simulink model "HANcoder_E407_TTA_Controller_v4_5"  (R2018b)
settings: Solver=FixedStepDiscrete  StartTime=0.0  StopTime=1  FixedStep=0.01  RelTol=1e-3
PreLoadFcn:
  | librarySetup
  | eval([bdroot,'_startup']) %Calling [modelName]_startup.m
values from neighbouring files (symbols this model uses):
  Backup_Board = 0    [HANcoder_E407_TTA_Controller_v3_5_startup.m]    (also in HANcoder_E407_TTA_Controller_v4_6_startup.m; HANcoder_E407_TTA_Controller_v4_7_startup.m; HANcoder_E407_TTA_Controller_v4_startup.m)
  basic_cycle_duration_bc0 = TM_Reset_Board   + COMP_duration    (= 212)    [HANcoder_E407_TTA_Controller_v3_5_startup.m]    (also in HANcoder_E407_TTA_Controller_v4_6_startup.m; HANcoder_E407_TTA_Controller_v4_7_startup.m; HANcoder_E407_TTA_Controller_v4_startup.m)
  basic_cycle_duration_bc1 = TM_Reset_Var_bc1 + COMP_duration    (= 288)    [HANcoder_E407_TTA_Controller_v3_5_startup.m]    (also in HANcoder_E407_TTA_Controller_v4_6_startup.m = 332; HANcoder_E407_TTA_Controller_v4_7_startup.m = 372; HANcoder_E407_TTA_Controller_v4_startup.m = 332)
  comm_delay_estimation1 = round(comm_delay_measured1*hardware_granularity/frequency_IRQ)    [HANcoder_E407_TTA_Controller_v3_5_startup.m]    (also in HANcoder_E407_TTA_Controller_v4_6_startup.m; HANcoder_E407_TTA_Controller_v4_7_startup.m; HANcoder_E407_TTA_Controller_v4_startup.m)
  comm_delay_estimation2 = round(comm_delay_measured2*hardware_granularity/frequency_IRQ)    [HANcoder_E407_TTA_Controller_v3_5_startup.m]    (also in HANcoder_E407_TTA_Controller_v4_6_startup.m; HANcoder_E407_TTA_Controller_v4_7_startup.m; HANcoder_E407_TTA_Controller_v4_startup.m)
  COMM_Period = 40    [HANcoder_E407_TTA_Controller_v3_5_startup.m]    (also in HANcoder_E407_TTA_Controller_v4_6_startup.m; HANcoder_E407_TTA_Controller_v4_7_startup.m; HANcoder_E407_TTA_Controller_v4_startup.m)
  COMM_Phase1 = Simulink.Parameter    [HANcoder_E407_TTA_Controller_v3_5_startup.m]    (also in HANcoder_E407_TTA_Controller_v4_6_startup.m; HANcoder_E407_TTA_Controller_v4_7_startup.m; HANcoder_E407_TTA_Controller_v4_startup.m)
  COMM_Phase2 = Simulink.Parameter    [HANcoder_E407_TTA_Controller_v3_5_startup.m]    (also in HANcoder_E407_TTA_Controller_v4_6_startup.m; HANcoder_E407_TTA_Controller_v4_7_startup.m; HANcoder_E407_TTA_Controller_v4_startup.m)
  COMM_Phase_init1 = Simulink.Parameter    [HANcoder_E407_TTA_Controller_v3_5_startup.m]    (also in HANcoder_E407_TTA_Controller_v4_6_startup.m; HANcoder_E407_TTA_Controller_v4_7_startup.m; HANcoder_E407_TTA_Controller_v4_startup.m)
  COMM_Phase_init2 = Simulink.Parameter    [HANcoder_E407_TTA_Controller_v3_5_startup.m]    (also in HANcoder_E407_TTA_Controller_v4_6_startup.m; HANcoder_E407_TTA_Controller_v4_7_startup.m; HANcoder_E407_TTA_Controller_v4_startup.m)
  COMP_duration = 4    [HANcoder_E407_TTA_Controller_v3_5_startup.m]    (also in HANcoder_E407_TTA_Controller_v4_6_startup.m; HANcoder_E407_TTA_Controller_v4_7_startup.m; HANcoder_E407_TTA_Controller_v4_startup.m)
  Controller1_Board = 1    [HANcoder_E407_TTA_Controller_v3_5_startup.m]    (also in HANcoder_E407_TTA_Controller_v4_6_startup.m; HANcoder_E407_TTA_Controller_v4_7_startup.m; HANcoder_E407_TTA_Controller_v4_startup.m)
  Controller2_Board = 2    [HANcoder_E407_TTA_Controller_v3_5_startup.m]    (also in HANcoder_E407_TTA_Controller_v4_6_startup.m; HANcoder_E407_TTA_Controller_v4_7_startup.m; HANcoder_E407_TTA_Controller_v4_startup.m)
  Controller3_Board = 3    [HANcoder_E407_TTA_Controller_v3_5_startup.m]    (also in HANcoder_E407_TTA_Controller_v4_6_startup.m; HANcoder_E407_TTA_Controller_v4_7_startup.m; HANcoder_E407_TTA_Controller_v4_startup.m)
  delta_a_set = Simulink.Parameter    [HANcoder_E407_TTA_Controller_v3_5_startup.m]    (also in HANcoder_E407_TTA_Controller_v4_6_startup.m; HANcoder_E407_TTA_Controller_v4_7_startup.m; HANcoder_E407_TTA_Controller_v4_startup.m)
  delta_f_set = Simulink.Parameter    [HANcoder_E407_TTA_Controller_v3_5_startup.m]    (also in HANcoder_E407_TTA_Controller_v4_6_startup.m; HANcoder_E407_TTA_Controller_v4_7_startup.m; HANcoder_E407_TTA_Controller_v4_startup.m)
  delta_max = 1    [HANcoder_E407_TTA_Controller_v3_5_startup.m]    (also in HANcoder_E407_TTA_Controller_v4_6_startup.m; HANcoder_E407_TTA_Controller_v4_7_startup.m; HANcoder_E407_TTA_Controller_v4_startup.m)
  delta_min = -1    [HANcoder_E407_TTA_Controller_v3_5_startup.m]    (also in HANcoder_E407_TTA_Controller_v4_6_startup.m; HANcoder_E407_TTA_Controller_v4_7_startup.m; HANcoder_E407_TTA_Controller_v4_startup.m)
  delta_precision = 6    [HANcoder_E407_TTA_Controller_v3_5_startup.m]    (also in HANcoder_E407_TTA_Controller_v4_6_startup.m; HANcoder_E407_TTA_Controller_v4_7_startup.m; HANcoder_E407_TTA_Controller_v4_startup.m)
  e_width = 0.1    [HANcoder_E407_TTA_Controller_v3_5_startup.m]    (also in HANcoder_E407_TTA_Controller_v4_6_startup.m; HANcoder_E407_TTA_Controller_v4_7_startup.m; HANcoder_E407_TTA_Controller_v4_startup.m)
  frequency_IRQ = 100    [HANcoder_E407_2xCAN_TEST_startup.m]    (also in HANcoder_E407_TTA_Controller_v3_5_startup.m; HANcoder_E407_TTA_Controller_v4_6_startup.m; HANcoder_E407_TTA_Controller_v4_7_startup.m; HANcoder_E407_TTA_Controller_v4_startup.m)
  HANtuneOverride = Simulink.Parameter    [HANcoder_E407_2xCAN_TEST_startup.m]    (also in HANcoder_E407_TTA_Controller_v3_5_startup.m; HANcoder_E407_TTA_Controller_v4_6_startup.m; HANcoder_E407_TTA_Controller_v4_7_startup.m; HANcoder_E407_TTA_Controller_v4_startup.m)
  hardware_granularity = 1000000    [HANcoder_E407_2xCAN_TEST_startup.m]    (also in HANcoder_E407_TTA_Controller_v3_5_startup.m; HANcoder_E407_TTA_Controller_v4_6_startup.m; HANcoder_E407_TTA_Controller_v4_7_startup.m; HANcoder_E407_TTA_Controller_v4_startup.m)
  I_a = 2.25    [HANcoder_E407_TTA_Controller_v3_5_startup.m]    (also in HANcoder_E407_TTA_Controller_v4_6_startup.m; HANcoder_E407_TTA_Controller_v4_7_startup.m; HANcoder_E407_TTA_Controller_v4_startup.m)
  I_f = 2.25    [HANcoder_E407_TTA_Controller_v3_5_startup.m]    (also in HANcoder_E407_TTA_Controller_v4_6_startup.m; HANcoder_E407_TTA_Controller_v4_7_startup.m; HANcoder_E407_TTA_Controller_v4_startup.m)
  idle_time_init = basic_cycle_duration_bc0 + basic_cycle_duration_bc1    (= 500)    [HANcoder_E407_TTA_Controller_v3_5_startup.m]    (also in HANcoder_E407_TTA_Controller_v4_6_startup.m = 544; HANcoder_E407_TTA_Controller_v4_7_startup.m = 584; HANcoder_E407_TTA_Controller_v4_startup.m = 544)
  Input_Gen_Board = 4    [HANcoder_E407_TTA_Controller_v3_5_startup.m]    (also in HANcoder_E407_TTA_Controller_v4_6_startup.m; HANcoder_E407_TTA_Controller_v4_7_startup.m; HANcoder_E407_TTA_Controller_v4_startup.m)
  LA_Clock_Gr = 1    [HANcoder_E407_TTA_Controller_v3_5_startup.m]    (also in HANcoder_E407_TTA_Controller_v4_6_startup.m; HANcoder_E407_TTA_Controller_v4_7_startup.m; HANcoder_E407_TTA_Controller_v4_startup.m)
  LA_COMM_dly = 1    [HANcoder_E407_TTA_Controller_v3_5_startup.m]    (also in HANcoder_E407_TTA_Controller_v4_6_startup.m; HANcoder_E407_TTA_Controller_v4_7_startup.m; HANcoder_E407_TTA_Controller_v4_startup.m)
  LA_COMM_Err = 1    [HANcoder_E407_TTA_Controller_v3_5_startup.m]    (also in HANcoder_E407_TTA_Controller_v4_6_startup.m; HANcoder_E407_TTA_Controller_v4_7_startup.m; HANcoder_E407_TTA_Controller_v4_startup.m)
  LA_E_Desync = 1    [HANcoder_E407_TTA_Controller_v3_5_startup.m]    (also in HANcoder_E407_TTA_Controller_v4_6_startup.m; HANcoder_E407_TTA_Controller_v4_7_startup.m; HANcoder_E407_TTA_Controller_v4_startup.m)
  LA_MEX_Flag = 1    [HANcoder_E407_TTA_Controller_v3_5_startup.m]    (also in HANcoder_E407_TTA_Controller_v4_6_startup.m; HANcoder_E407_TTA_Controller_v4_7_startup.m; HANcoder_E407_TTA_Controller_v4_startup.m)
  LA_Task_Act = 1    [HANcoder_E407_TTA_Controller_v3_5_startup.m]    (also in HANcoder_E407_TTA_Controller_v4_6_startup.m; HANcoder_E407_TTA_Controller_v4_7_startup.m; HANcoder_E407_TTA_Controller_v4_startup.m)
  m_v = 100.0    (= 100)    [HANcoder_E407_TTA_Controller_v3_5_startup.m]    (also in HANcoder_E407_TTA_Controller_v4_6_startup.m; HANcoder_E407_TTA_Controller_v4_7_startup.m; HANcoder_E407_TTA_Controller_v4_startup.m)
  Master_Role = 1    [HANcoder_E407_TTA_Controller_v3_5_startup.m]    (also in HANcoder_E407_TTA_Controller_v4_6_startup.m; HANcoder_E407_TTA_Controller_v4_7_startup.m; HANcoder_E407_TTA_Controller_v4_startup.m)
  matrix_cycle_duration = basic_cycle_duration_bc0 + basic_cycle_duration_bc1    (= 500)    [HANcoder_E407_TTA_Controller_v3_5_startup.m]    (also in HANcoder_E407_TTA_Controller_v4_6_startup.m = 544; HANcoder_E407_TTA_Controller_v4_7_startup.m = 584; HANcoder_E407_TTA_Controller_v4_startup.m = 544)
  matrix_rows = 2    [HANcoder_E407_TTA_Controller_v3_5_startup.m]    (also in HANcoder_E407_TTA_Controller_v4_6_startup.m; HANcoder_E407_TTA_Controller_v4_7_startup.m; HANcoder_E407_TTA_Controller_v4_startup.m)
  max_desync = 15    [HANcoder_E407_TTA_Controller_v3_5_startup.m]    (also in HANcoder_E407_TTA_Controller_v4_6_startup.m; HANcoder_E407_TTA_Controller_v4_7_startup.m = 30; HANcoder_E407_TTA_Controller_v4_startup.m)
  max_num_msgs_CAN1 = 2^Tx_bit_number-1    (= 7)    [HANcoder_E407_TTA_Controller_v3_5_startup.m]    (also in HANcoder_E407_TTA_Controller_v4_6_startup.m = 15; HANcoder_E407_TTA_Controller_v4_7_startup.m = 15; HANcoder_E407_TTA_Controller_v4_startup.m)
  max_num_msgs_CAN2 = max_num_msgs_CAN1    (= 7)    [HANcoder_E407_TTA_Controller_v3_5_startup.m]    (also in HANcoder_E407_TTA_Controller_v4_6_startup.m = 15; HANcoder_E407_TTA_Controller_v4_7_startup.m = 15; HANcoder_E407_TTA_Controller_v4_startup.m)
  min_desync = (-1)*max_desync    (= -15)    [HANcoder_E407_TTA_Controller_v3_5_startup.m]    (also in HANcoder_E407_TTA_Controller_v4_6_startup.m; HANcoder_E407_TTA_Controller_v4_7_startup.m = -30; HANcoder_E407_TTA_Controller_v4_startup.m)
  OutControl1_ID = 23    [HANcoder_E407_TTA_Controller_v3_5_startup.m]    (also in HANcoder_E407_TTA_Controller_v4_6_startup.m; HANcoder_E407_TTA_Controller_v4_7_startup.m; HANcoder_E407_TTA_Controller_v4_startup.m)
  OutControl2_ID = 24    [HANcoder_E407_TTA_Controller_v3_5_startup.m]    (also in HANcoder_E407_TTA_Controller_v4_6_startup.m; HANcoder_E407_TTA_Controller_v4_7_startup.m; HANcoder_E407_TTA_Controller_v4_startup.m)
  OutEmulator_ID = 25    [HANcoder_E407_TTA_Controller_v3_5_startup.m]    (also in HANcoder_E407_TTA_Controller_v4_6_startup.m = 26; HANcoder_E407_TTA_Controller_v4_7_startup.m = 26; HANcoder_E407_TTA_Controller_v4_startup.m)
  OutMaster_ID = 25    [HANcoder_E407_TTA_Controller_v4_6_startup.m]    (also in HANcoder_E407_TTA_Controller_v4_7_startup.m; HANcoder_E407_TTA_Controller_v4_startup.m = 26)
  R_al = 0.10    (= 0.1)    [HANcoder_E407_TTA_Controller_v3_5_startup.m]    (also in HANcoder_E407_TTA_Controller_v4_6_startup.m; HANcoder_E407_TTA_Controller_v4_7_startup.m; HANcoder_E407_TTA_Controller_v4_startup.m)
  R_ar = 0.10    (= 0.1)    [HANcoder_E407_TTA_Controller_v3_5_startup.m]    (also in HANcoder_E407_TTA_Controller_v4_6_startup.m; HANcoder_E407_TTA_Controller_v4_7_startup.m; HANcoder_E407_TTA_Controller_v4_startup.m)
  R_fl = 0.10    (= 0.1)    [HANcoder_E407_TTA_Controller_v3_5_startup.m]    (also in HANcoder_E407_TTA_Controller_v4_6_startup.m; HANcoder_E407_TTA_Controller_v4_7_startup.m; HANcoder_E407_TTA_Controller_v4_startup.m)
  R_fr = 0.10    (= 0.1)    [HANcoder_E407_TTA_Controller_v3_5_startup.m]    (also in HANcoder_E407_TTA_Controller_v4_6_startup.m; HANcoder_E407_TTA_Controller_v4_7_startup.m; HANcoder_E407_TTA_Controller_v4_startup.m)
  script_run = Simulink.Parameter    [HANcoder_E407_TTA_Controller_v3_5_startup.m]    (also in HANcoder_E407_TTA_Controller_v4_6_startup.m; HANcoder_E407_TTA_Controller_v4_7_startup.m; HANcoder_E407_TTA_Controller_v4_startup.m)
  SensorValues_ID = 22    [HANcoder_E407_TTA_Controller_v3_5_startup.m]    (also in HANcoder_E407_TTA_Controller_v4_6_startup.m; HANcoder_E407_TTA_Controller_v4_7_startup.m; HANcoder_E407_TTA_Controller_v4_startup.m)
  SetValues_ID = 21    [HANcoder_E407_TTA_Controller_v3_5_startup.m]    (also in HANcoder_E407_TTA_Controller_v4_6_startup.m; HANcoder_E407_TTA_Controller_v4_7_startup.m; HANcoder_E407_TTA_Controller_v4_startup.m)
  Slave_Role = 2    [HANcoder_E407_TTA_Controller_v3_5_startup.m]    (also in HANcoder_E407_TTA_Controller_v4_6_startup.m; HANcoder_E407_TTA_Controller_v4_7_startup.m; HANcoder_E407_TTA_Controller_v4_startup.m)
  speed_k_d = Simulink.Parameter    [HANcoder_E407_TTA_Controller_v3_5_startup.m]    (also in HANcoder_E407_TTA_Controller_v4_6_startup.m; HANcoder_E407_TTA_Controller_v4_7_startup.m; HANcoder_E407_TTA_Controller_v4_startup.m)
  speed_k_i = Simulink.Parameter    [HANcoder_E407_TTA_Controller_v3_5_startup.m]    (also in HANcoder_E407_TTA_Controller_v4_6_startup.m; HANcoder_E407_TTA_Controller_v4_7_startup.m; HANcoder_E407_TTA_Controller_v4_startup.m)
  speed_k_p = Simulink.Parameter    [HANcoder_E407_TTA_Controller_v3_5_startup.m]    (also in HANcoder_E407_TTA_Controller_v4_6_startup.m; HANcoder_E407_TTA_Controller_v4_7_startup.m; HANcoder_E407_TTA_Controller_v4_startup.m)
  speed_max = 10    [HANcoder_E407_TTA_Controller_v3_5_startup.m]    (also in HANcoder_E407_TTA_Controller_v4_6_startup.m; HANcoder_E407_TTA_Controller_v4_7_startup.m; HANcoder_E407_TTA_Controller_v4_startup.m)
  speed_min = -10    [HANcoder_E407_TTA_Controller_v3_5_startup.m]    (also in HANcoder_E407_TTA_Controller_v4_6_startup.m; HANcoder_E407_TTA_Controller_v4_7_startup.m; HANcoder_E407_TTA_Controller_v4_startup.m)
  speed_precision = 3    [HANcoder_E407_TTA_Controller_v3_5_startup.m]    (also in HANcoder_E407_TTA_Controller_v4_6_startup.m; HANcoder_E407_TTA_Controller_v4_7_startup.m; HANcoder_E407_TTA_Controller_v4_startup.m)
  Sync_ID = 1    [HANcoder_E407_TTA_Controller_v3_5_startup.m]    (also in HANcoder_E407_TTA_Controller_v4_6_startup.m; HANcoder_E407_TTA_Controller_v4_7_startup.m; HANcoder_E407_TTA_Controller_v4_startup.m)
  tau_max = 5    [HANcoder_E407_TTA_Controller_v3_5_startup.m]    (also in HANcoder_E407_TTA_Controller_v4_6_startup.m; HANcoder_E407_TTA_Controller_v4_7_startup.m; HANcoder_E407_TTA_Controller_v4_startup.m)
  tau_min = -5    [HANcoder_E407_TTA_Controller_v3_5_startup.m]    (also in HANcoder_E407_TTA_Controller_v4_6_startup.m; HANcoder_E407_TTA_Controller_v4_7_startup.m; HANcoder_E407_TTA_Controller_v4_startup.m)
  tau_range = abs(tau_max) + abs(tau_min)    [HANcoder_E407_TTA_Controller_v3_5_startup.m]    (also in HANcoder_E407_TTA_Controller_v4_6_startup.m; HANcoder_E407_TTA_Controller_v4_7_startup.m; HANcoder_E407_TTA_Controller_v4_startup.m)
  theta_max = (speed_max/R_fr)*matrix_cycle_duration*frequency_IRQ/hardware_granularity    (= 5)    [HANcoder_E407_TTA_Controller_v3_5_startup.m]    (also in HANcoder_E407_TTA_Controller_v4_6_startup.m = 5.44; HANcoder_E407_TTA_Controller_v4_7_startup.m = 5.84; HANcoder_E407_TTA_Controller_v4_startup.m = 5.44)
  theta_min = (-1)*theta_max    (= -5)    [HANcoder_E407_TTA_Controller_v3_5_startup.m]    (also in HANcoder_E407_TTA_Controller_v4_6_startup.m = -5.44; HANcoder_E407_TTA_Controller_v4_7_startup.m = -5.84; HANcoder_E407_TTA_Controller_v4_startup.m = -5.44)
  theta_precision = 7-(fix(log2(theta_max))+1)    [HANcoder_E407_TTA_Controller_v3_5_startup.m]    (also in HANcoder_E407_TTA_Controller_v4_6_startup.m; HANcoder_E407_TTA_Controller_v4_7_startup.m; HANcoder_E407_TTA_Controller_v4_startup.m)
  Tl_a = 0.6    [HANcoder_E407_TTA_Controller_v3_5_startup.m]    (also in HANcoder_E407_TTA_Controller_v4_6_startup.m; HANcoder_E407_TTA_Controller_v4_7_startup.m; HANcoder_E407_TTA_Controller_v4_startup.m)
  Tl_f = 0.6    [HANcoder_E407_TTA_Controller_v3_5_startup.m]    (also in HANcoder_E407_TTA_Controller_v4_6_startup.m; HANcoder_E407_TTA_Controller_v4_7_startup.m; HANcoder_E407_TTA_Controller_v4_startup.m)
  TM_Check_Output_Control1 = TM_COMM_Output_Control1 + COMM_duration    (= 188)    [HANcoder_E407_TTA_Controller_v3_5_startup.m]    (also in HANcoder_E407_TTA_Controller_v4_6_startup.m; HANcoder_E407_TTA_Controller_v4_7_startup.m; HANcoder_E407_TTA_Controller_v4_startup.m)
  TM_Check_Output_Control2 = TM_COMM_Output_Control2 + COMM_duration    (= 232)    [HANcoder_E407_TTA_Controller_v3_5_startup.m]    (also in HANcoder_E407_TTA_Controller_v4_6_startup.m; HANcoder_E407_TTA_Controller_v4_7_startup.m; HANcoder_E407_TTA_Controller_v4_startup.m)
  TM_Check_Output_Emulator = TM_COMM_Output_Emulator + COMM_duration    (= 280)    [HANcoder_E407_TTA_Controller_v3_5_startup.m]    (also in HANcoder_E407_TTA_Controller_v4_6_startup.m = 320; HANcoder_E407_TTA_Controller_v4_7_startup.m = 360; HANcoder_E407_TTA_Controller_v4_startup.m = 320)
  TM_Check_Output_Emulator_2 = TM_Check_Output_Emulator + 2    (= 282)    [HANcoder_E407_TTA_Controller_v3_5_startup.m]    (also in HANcoder_E407_TTA_Controller_v4_6_startup.m = 322; HANcoder_E407_TTA_Controller_v4_7_startup.m = 362; HANcoder_E407_TTA_Controller_v4_startup.m = 322)
  TM_Check_Output_Emulator_3 = TM_Check_Output_Emulator_2 + 2    (= 324)    [HANcoder_E407_TTA_Controller_v4_6_startup.m]    (also in HANcoder_E407_TTA_Controller_v4_7_startup.m = 364; HANcoder_E407_TTA_Controller_v4_startup.m)
  TM_Check_Sensor_Values = TM_COMM_Sensor_Values + COMM_duration    (= 132)    [HANcoder_E407_TTA_Controller_v3_5_startup.m]    (also in HANcoder_E407_TTA_Controller_v4_6_startup.m; HANcoder_E407_TTA_Controller_v4_7_startup.m; HANcoder_E407_TTA_Controller_v4_startup.m)
  TM_Check_Sensor_Values_2 = TM_Check_Sensor_Values + 2    (= 134)    [HANcoder_E407_TTA_Controller_v3_5_startup.m]    (also in HANcoder_E407_TTA_Controller_v4_6_startup.m; HANcoder_E407_TTA_Controller_v4_7_startup.m; HANcoder_E407_TTA_Controller_v4_startup.m)
  TM_Check_Set_Values = TM_COMM_Set_Values + COMM_duration    (= 88)    [HANcoder_E407_TTA_Controller_v3_5_startup.m]    (also in HANcoder_E407_TTA_Controller_v4_6_startup.m; HANcoder_E407_TTA_Controller_v4_7_startup.m; HANcoder_E407_TTA_Controller_v4_startup.m)
  TM_Check_Set_Values_2 = TM_Check_Set_Values + 2    (= 90)    [HANcoder_E407_TTA_Controller_v3_5_startup.m]    (also in HANcoder_E407_TTA_Controller_v4_6_startup.m; HANcoder_E407_TTA_Controller_v4_7_startup.m; HANcoder_E407_TTA_Controller_v4_startup.m)
  TM_Check_Sync = TM_COMM_Sync   + COMM_duration    (= 40)    [HANcoder_E407_TTA_Controller_v3_5_startup.m]    (also in HANcoder_E407_TTA_Controller_v4_6_startup.m; HANcoder_E407_TTA_Controller_v4_7_startup.m; HANcoder_E407_TTA_Controller_v4_startup.m)
  TM_Check_TOuts = TM_Count_Vote3 + COMP_duration    (= 196)    [HANcoder_E407_TTA_Controller_v3_5_startup.m]    (also in HANcoder_E407_TTA_Controller_v4_6_startup.m; HANcoder_E407_TTA_Controller_v4_7_startup.m; HANcoder_E407_TTA_Controller_v4_startup.m)
  TM_Check_Vote1 = TM_COMM_Vote1  + COMM_duration    (= 92)    [HANcoder_E407_TTA_Controller_v3_5_startup.m]    (also in HANcoder_E407_TTA_Controller_v4_6_startup.m; HANcoder_E407_TTA_Controller_v4_7_startup.m; HANcoder_E407_TTA_Controller_v4_startup.m)
  TM_Check_Vote2 = TM_COMM_Vote2  + COMM_duration    (= 140)    [HANcoder_E407_TTA_Controller_v3_5_startup.m]    (also in HANcoder_E407_TTA_Controller_v4_6_startup.m; HANcoder_E407_TTA_Controller_v4_7_startup.m; HANcoder_E407_TTA_Controller_v4_startup.m)
  TM_Check_Vote2_2 = TM_Check_Vote2 + 2    (= 142)    [HANcoder_E407_TTA_Controller_v3_5_startup.m]    (also in HANcoder_E407_TTA_Controller_v4_6_startup.m; HANcoder_E407_TTA_Controller_v4_7_startup.m; HANcoder_E407_TTA_Controller_v4_startup.m)
  TM_Check_Vote3 = TM_COMM_Vote3  + COMM_duration    (= 188)    [HANcoder_E407_TTA_Controller_v3_5_startup.m]    (also in HANcoder_E407_TTA_Controller_v4_6_startup.m; HANcoder_E407_TTA_Controller_v4_7_startup.m; HANcoder_E407_TTA_Controller_v4_startup.m)
  TM_COMM_Output_Control1 = TM_Velocity + COMP_duration    (= 148)    [HANcoder_E407_TTA_Controller_v3_5_startup.m]    (also in HANcoder_E407_TTA_Controller_v4_6_startup.m; HANcoder_E407_TTA_Controller_v4_7_startup.m; HANcoder_E407_TTA_Controller_v4_startup.m)
  TM_COMM_Output_Control2 = TM_Check_Output_Control1 + COMP_duration    (= 192)    [HANcoder_E407_TTA_Controller_v3_5_startup.m]    (also in HANcoder_E407_TTA_Controller_v4_6_startup.m; HANcoder_E407_TTA_Controller_v4_7_startup.m; HANcoder_E407_TTA_Controller_v4_startup.m)
  TM_COMM_Output_Emulator = TM_TMR + COMP_duration    (= 240)    [HANcoder_E407_TTA_Controller_v3_5_startup.m]    (also in HANcoder_E407_TTA_Controller_v4_6_startup.m = 280; HANcoder_E407_TTA_Controller_v4_7_startup.m = 320; HANcoder_E407_TTA_Controller_v4_startup.m = 280)
  TM_COMM_Output_Master = TM_Check_Output_Control2 + COMM_duration    (= 272)    [HANcoder_E407_TTA_Controller_v4_6_startup.m]    (also in HANcoder_E407_TTA_Controller_v4_7_startup.m; HANcoder_E407_TTA_Controller_v4_startup.m)
  TM_COMM_Sensor_Values = TM_Check_Set_Values + COMP_duration    (= 92)    [HANcoder_E407_TTA_Controller_v3_5_startup.m]    (also in HANcoder_E407_TTA_Controller_v4_6_startup.m; HANcoder_E407_TTA_Controller_v4_7_startup.m; HANcoder_E407_TTA_Controller_v4_startup.m)
  TM_COMM_Set_Values = TM_Update_LT + COMP_duration    (= 48)    [HANcoder_E407_TTA_Controller_v3_5_startup.m]    (also in HANcoder_E407_TTA_Controller_v4_6_startup.m; HANcoder_E407_TTA_Controller_v4_7_startup.m; HANcoder_E407_TTA_Controller_v4_startup.m)
  TM_COMM_Sync = basic_cycle_start    (= 0)    [HANcoder_E407_TTA_Controller_v3_5_startup.m]    (also in HANcoder_E407_TTA_Controller_v4_6_startup.m; HANcoder_E407_TTA_Controller_v4_7_startup.m; HANcoder_E407_TTA_Controller_v4_startup.m)
  TM_COMM_Vote1 = TM_Vote_Dec    + COMP_duration    (= 52)    [HANcoder_E407_TTA_Controller_v3_5_startup.m]    (also in HANcoder_E407_TTA_Controller_v4_6_startup.m; HANcoder_E407_TTA_Controller_v4_7_startup.m; HANcoder_E407_TTA_Controller_v4_startup.m)
  TM_COMM_Vote2 = TM_Count_Vote1 + COMP_duration    (= 100)    [HANcoder_E407_TTA_Controller_v3_5_startup.m]    (also in HANcoder_E407_TTA_Controller_v4_6_startup.m; HANcoder_E407_TTA_Controller_v4_7_startup.m; HANcoder_E407_TTA_Controller_v4_startup.m)
  TM_COMM_Vote3 = TM_Count_Vote2 + COMP_duration    (= 148)    [HANcoder_E407_TTA_Controller_v3_5_startup.m]    (also in HANcoder_E407_TTA_Controller_v4_6_startup.m; HANcoder_E407_TTA_Controller_v4_7_startup.m; HANcoder_E407_TTA_Controller_v4_startup.m)
  TM_Count_Vote1 = TM_Check_Vote1 + COMP_duration    (= 96)    [HANcoder_E407_TTA_Controller_v3_5_startup.m]    (also in HANcoder_E407_TTA_Controller_v4_6_startup.m; HANcoder_E407_TTA_Controller_v4_7_startup.m; HANcoder_E407_TTA_Controller_v4_startup.m)
  TM_Count_Vote2 = TM_Check_Vote2 + COMP_duration    (= 144)    [HANcoder_E407_TTA_Controller_v3_5_startup.m]    (also in HANcoder_E407_TTA_Controller_v4_6_startup.m; HANcoder_E407_TTA_Controller_v4_7_startup.m; HANcoder_E407_TTA_Controller_v4_startup.m)
  TM_Count_Vote3 = TM_Check_Vote3 + COMP_duration    (= 192)    [HANcoder_E407_TTA_Controller_v3_5_startup.m]    (also in HANcoder_E407_TTA_Controller_v4_6_startup.m; HANcoder_E407_TTA_Controller_v4_7_startup.m; HANcoder_E407_TTA_Controller_v4_startup.m)
  TM_Data_bc0 = TM_COMM_Sync    (= 0)    [HANcoder_E407_TTA_Controller_v3_5_startup.m]    (also in HANcoder_E407_TTA_Controller_v4_6_startup.m; HANcoder_E407_TTA_Controller_v4_7_startup.m; HANcoder_E407_TTA_Controller_v4_startup.m)
  TM_Data_bc1 = TM_Data_bc0(1:4)    [HANcoder_E407_TTA_Controller_v3_5_startup.m]    (also in HANcoder_E407_TTA_Controller_v4_6_startup.m; HANcoder_E407_TTA_Controller_v4_7_startup.m; HANcoder_E407_TTA_Controller_v4_startup.m)
  TM_New_Master = TM_Check_TOuts + COMP_duration    (= 200)    [HANcoder_E407_TTA_Controller_v3_5_startup.m]    (also in HANcoder_E407_TTA_Controller_v4_6_startup.m; HANcoder_E407_TTA_Controller_v4_7_startup.m; HANcoder_E407_TTA_Controller_v4_startup.m)
  TM_Reset_Board = TM_Reset_Var   + COMP_duration    (= 208)    [HANcoder_E407_TTA_Controller_v3_5_startup.m]    (also in HANcoder_E407_TTA_Controller_v4_6_startup.m; HANcoder_E407_TTA_Controller_v4_7_startup.m; HANcoder_E407_TTA_Controller_v4_startup.m)
  TM_Reset_Var = TM_New_Master  + COMP_duration    (= 204)    [HANcoder_E407_TTA_Controller_v3_5_startup.m]    (also in HANcoder_E407_TTA_Controller_v4_6_startup.m; HANcoder_E407_TTA_Controller_v4_7_startup.m; HANcoder_E407_TTA_Controller_v4_startup.m)
  TM_Reset_Var_bc1 = TM_Check_Output_Emulator + COMP_duration    (= 284)    [HANcoder_E407_TTA_Controller_v3_5_startup.m]    (also in HANcoder_E407_TTA_Controller_v4_6_startup.m = 328; HANcoder_E407_TTA_Controller_v4_7_startup.m = 368; HANcoder_E407_TTA_Controller_v4_startup.m = 328)
  TM_Reset_Var_bc1_2 = TM_Reset_Var_bc1 + 2    (= 286)    [HANcoder_E407_TTA_Controller_v3_5_startup.m]    (also in HANcoder_E407_TTA_Controller_v4_6_startup.m = 330; HANcoder_E407_TTA_Controller_v4_7_startup.m = 370; HANcoder_E407_TTA_Controller_v4_startup.m = 330)
  TM_Steer = TM_Check_Sensor_Values + COMP_duration    (= 136)    [HANcoder_E407_TTA_Controller_v3_5_startup.m]    (also in HANcoder_E407_TTA_Controller_v4_6_startup.m; HANcoder_E407_TTA_Controller_v4_7_startup.m; HANcoder_E407_TTA_Controller_v4_startup.m)
  TM_TMR = TM_Check_Output_Control2 + COMP_duration    (= 236)    [HANcoder_E407_TTA_Controller_v3_5_startup.m]    (also in HANcoder_E407_TTA_Controller_v4_6_startup.m = 276; HANcoder_E407_TTA_Controller_v4_7_startup.m = 316; HANcoder_E407_TTA_Controller_v4_startup.m = 276)
  TM_TMR_2 = TM_TMR + 1    (= 237)    [HANcoder_E407_TTA_Controller_v3_5_startup.m]    (also in HANcoder_E407_TTA_Controller_v4_6_startup.m = 277; HANcoder_E407_TTA_Controller_v4_7_startup.m = 317; HANcoder_E407_TTA_Controller_v4_startup.m = 277)
  TM_TMR_3 = TM_TMR + 3    (= 239)    [HANcoder_E407_TTA_Controller_v3_5_startup.m]    (also in HANcoder_E407_TTA_Controller_v4_6_startup.m = 279; HANcoder_E407_TTA_Controller_v4_7_startup.m = 319; HANcoder_E407_TTA_Controller_v4_startup.m = 279)
  TM_Torque = TM_Steer + COMP_duration    (= 140)    [HANcoder_E407_TTA_Controller_v3_5_startup.m]    (also in HANcoder_E407_TTA_Controller_v4_6_startup.m; HANcoder_E407_TTA_Controller_v4_7_startup.m; HANcoder_E407_TTA_Controller_v4_startup.m)
  TM_Type_bc0 = COMM    (= 0)    [HANcoder_E407_TTA_Controller_v3_5_startup.m]    (also in HANcoder_E407_TTA_Controller_v4_6_startup.m; HANcoder_E407_TTA_Controller_v4_7_startup.m; HANcoder_E407_TTA_Controller_v4_startup.m)
  TM_Type_bc1 = TM_Type_bc0(1:4)    [HANcoder_E407_TTA_Controller_v3_5_startup.m]    (also in HANcoder_E407_TTA_Controller_v4_6_startup.m; HANcoder_E407_TTA_Controller_v4_7_startup.m; HANcoder_E407_TTA_Controller_v4_startup.m)
  TM_Update_LT = TM_Check_Sync  + COMP_duration    (= 44)    [HANcoder_E407_TTA_Controller_v3_5_startup.m]    (also in HANcoder_E407_TTA_Controller_v4_6_startup.m; HANcoder_E407_TTA_Controller_v4_7_startup.m; HANcoder_E407_TTA_Controller_v4_startup.m)
  TM_Update_LT_2 = TM_Update_LT   + 2    (= 46)    [HANcoder_E407_TTA_Controller_v3_5_startup.m]    (also in HANcoder_E407_TTA_Controller_v4_6_startup.m; HANcoder_E407_TTA_Controller_v4_7_startup.m; HANcoder_E407_TTA_Controller_v4_startup.m)
  TM_Velocity = TM_Torque + COMP_duration    (= 144)    [HANcoder_E407_TTA_Controller_v3_5_startup.m]    (also in HANcoder_E407_TTA_Controller_v4_6_startup.m; HANcoder_E407_TTA_Controller_v4_7_startup.m; HANcoder_E407_TTA_Controller_v4_startup.m)
  TM_Vote_Dec = TM_Update_LT   + COMP_duration    (= 48)    [HANcoder_E407_TTA_Controller_v3_5_startup.m]    (also in HANcoder_E407_TTA_Controller_v4_6_startup.m; HANcoder_E407_TTA_Controller_v4_7_startup.m; HANcoder_E407_TTA_Controller_v4_startup.m)
  TM_Vote_Dec_2 = TM_Vote_Dec    + 2    (= 50)    [HANcoder_E407_TTA_Controller_v3_5_startup.m]    (also in HANcoder_E407_TTA_Controller_v4_6_startup.m; HANcoder_E407_TTA_Controller_v4_7_startup.m; HANcoder_E407_TTA_Controller_v4_startup.m)
  torque_a_k_d = Simulink.Parameter    [HANcoder_E407_TTA_Controller_v3_5_startup.m]    (also in HANcoder_E407_TTA_Controller_v4_6_startup.m; HANcoder_E407_TTA_Controller_v4_7_startup.m; HANcoder_E407_TTA_Controller_v4_startup.m)
  torque_a_k_i = Simulink.Parameter    [HANcoder_E407_TTA_Controller_v3_5_startup.m]    (also in HANcoder_E407_TTA_Controller_v4_6_startup.m; HANcoder_E407_TTA_Controller_v4_7_startup.m; HANcoder_E407_TTA_Controller_v4_startup.m)
  torque_a_k_p = Simulink.Parameter    [HANcoder_E407_TTA_Controller_v3_5_startup.m]    (also in HANcoder_E407_TTA_Controller_v4_6_startup.m; HANcoder_E407_TTA_Controller_v4_7_startup.m; HANcoder_E407_TTA_Controller_v4_startup.m)
  torque_f_k_d = Simulink.Parameter    [HANcoder_E407_TTA_Controller_v3_5_startup.m]    (also in HANcoder_E407_TTA_Controller_v4_6_startup.m; HANcoder_E407_TTA_Controller_v4_7_startup.m; HANcoder_E407_TTA_Controller_v4_startup.m)
  torque_f_k_i = Simulink.Parameter    [HANcoder_E407_TTA_Controller_v3_5_startup.m]    (also in HANcoder_E407_TTA_Controller_v4_6_startup.m; HANcoder_E407_TTA_Controller_v4_7_startup.m; HANcoder_E407_TTA_Controller_v4_startup.m)
  ... (+7 more)
undefined symbols (not defined in the file or in its folder): A0, A1, A2, A3, A4, CON2, CON3, CON4, D10, D12, D13, D2, D3, D8, D9
libraries: hdlsllib x467, HANcoder_STM32_Target x30, simulink x3, simulink_extras x1
(part 43 of 80)

== system HANcoder_E407_TTA_Controller_v4_5/HANcoder STM32 Target - E407-STM32 algorithm/TTA CAN System/TTA System/Matrix Cycle Manager/Backup Board Matrix Cycle/Backup board basic cycle 1/COMP Task - MF/MF_load_msgs_3/uint8_2float6 ==
  precision : Inport
  value : Inport  Port=2
  Bit Shift : hdlsllib/Logic and Bit Operations/Bit Shift  mode=Shift Right Logical  N=7
      settings: SourceProductName=HDL Coder  SourceProductBaseCode=HD
  Bit Shift1 : hdlsllib/Logic and Bit Operations/Bit Shift  mode=Shift Left Logical  N=7
      settings: SourceProductName=HDL Coder  SourceProductBaseCode=HD
  Cast1 : DataTypeConversion  OutDataTypeStr=double
  Constant1 : Constant  Value=2
  Constant2 : Constant  Value=2
  Divide : Product  Inputs=*/
  Fix1 : Rounding  Operator=fix
  Gain : Gain  Gain=-1
  Gain1 : Gain  Gain=-1
  Minus : Sum  Inputs=-+
  Minus1 : Sum  Inputs=+-
  Minus2 : Sum
  Multiply : Product
  Multiply1 : Product
  Power : Math  Priority=5  Operator=pow  SaturateOnIntegerOverflow=on
  Power1 : Math  Priority=5  Operator=pow  SaturateOnIntegerOverflow=on
  Switch : Switch  Criteria=u2 > Threshold
  decoded : Outport
  wires:
  Bit Shift1/1 -> Minus/1
  [prec_pow] -> Multiply1/2
  [prec_pow] -> Divide/2
  Power1/1 -> [prec_pow]
  Constant2/1 -> Power1/1
  precision/1 -> [precision], Power1/2
  Cast1/1 -> Minus/2
  Divide/1 -> Fix1/1
  Switch/1 -> decoded/1
  Gain1/1 -> Switch/1
  Minus2/1 -> Switch/3, Gain1/1
  Multiply/1 -> Minus2/1
  [precision] -> Gain/1
  Power/1 -> Multiply/2
  Gain/1 -> Power/2
  Constant1/1 -> Power/1
  Minus1/1 -> Multiply/1
  Multiply1/1 -> Minus1/2
  Fix1/1 -> Multiply1/1, Minus2/2
  Minus/1 -> Minus1/1, Divide/1
  value/1 -> Bit Shift/1, Cast1/1
  Bit Shift/1 -> Switch/2, Bit Shift1/1

== system HANcoder_E407_TTA_Controller_v4_5/HANcoder STM32 Target - E407-STM32 algorithm/TTA CAN System/TTA System/Matrix Cycle Manager/Backup Board Matrix Cycle/Backup board basic cycle 1/COMP Task - MF/MF_load_msgs_3/uint8_2float7 ==
  precision : Inport
  value : Inport  Port=2
  Bit Shift : hdlsllib/Logic and Bit Operations/Bit Shift  mode=Shift Right Logical  N=7
      settings: SourceProductName=HDL Coder  SourceProductBaseCode=HD
  Bit Shift1 : hdlsllib/Logic and Bit Operations/Bit Shift  mode=Shift Left Logical  N=7
      settings: SourceProductName=HDL Coder  SourceProductBaseCode=HD
  Cast1 : DataTypeConversion  OutDataTypeStr=double
  Constant1 : Constant  Value=2
  Constant2 : Constant  Value=2
  Divide : Product  Inputs=*/
  Fix1 : Rounding  Operator=fix
  Gain : Gain  Gain=-1
  Gain1 : Gain  Gain=-1
  Minus : Sum  Inputs=-+
  Minus1 : Sum  Inputs=+-
  Minus2 : Sum
  Multiply : Product
  Multiply1 : Product
  Power : Math  Priority=5  Operator=pow  SaturateOnIntegerOverflow=on
  Power1 : Math  Priority=5  Operator=pow  SaturateOnIntegerOverflow=on
  Switch : Switch  Criteria=u2 > Threshold
  decoded : Outport
  wires:
  Bit Shift/1 -> Bit Shift1/1, Switch/2
  value/1 -> Cast1/1, Bit Shift/1
  Minus/1 -> Divide/1, Minus1/1
  Fix1/1 -> Minus2/2, Multiply1/1
  Multiply1/1 -> Minus1/2
  Minus1/1 -> Multiply/1
  Constant1/1 -> Power/1
  Gain/1 -> Power/2
  Power/1 -> Multiply/2
  [precision] -> Gain/1
  Multiply/1 -> Minus2/1
  Minus2/1 -> Gain1/1, Switch/3
  Gain1/1 -> Switch/1
  Switch/1 -> decoded/1
  Divide/1 -> Fix1/1
  Cast1/1 -> Minus/2
  precision/1 -> Power1/2, [precision]
  Constant2/1 -> Power1/1
  Power1/1 -> [prec_pow]
  [prec_pow] -> Divide/2
  [prec_pow] -> Multiply1/2
  Bit Shift1/1 -> Minus/1

== system HANcoder_E407_TTA_Controller_v4_5/HANcoder STM32 Target - E407-STM32 algorithm/TTA CAN System/TTA System/Matrix Cycle Manager/Backup Board Matrix Cycle/Backup board basic cycle 1/COMP Task - MF/MF_main/Agreement between Out1 and out3 ==
  Enable : EnablePort
  AND{,1..3} (4 alike) : Logic  IconShape=distinctive  AllPortsSameDT=off  OutDataTypeStr=boolean
  Constant{,1..7} (8 alike) : Constant  Value=tau_range
  Data Store Read : DataStoreRead  DataStoreName=tau_fr_out1
  Data Store Read1 : DataStoreRead  DataStoreName=tau_fl_out1
  Data Store Read2 : DataStoreRead  DataStoreName=tau_ar_out1
  Data Store Read3 : DataStoreRead  DataStoreName=tau_al_out1
  Data Store Read4 : DataStoreRead  DataStoreName=tau_fr_out3
  Data Store Read5 : DataStoreRead  DataStoreName=tau_fl_out3
  Data Store Read6 : DataStoreRead  DataStoreName=tau_ar_out3
  Data Store Read7 : DataStoreRead  DataStoreName=tau_al_out3
  Gain{,1..7} (8 alike) : Gain  Gain=e_width
  GreaterThan{,2,4,6} (4 alike) : RelationalOperator  OutDataTypeStr=boolean  RndMeth=Simplest
  GreaterThan{1,3,5,7} (4 alike) : RelationalOperator  Operator=<=  OutDataTypeStr=boolean  RndMeth=Simplest
  Plus{,2,4,6} (4 alike) : Sum
  Plus{1,3,5,7} (4 alike) : Sum  Inputs=+-
  tau_fr_agree : Outport  OutputWhenDisabled=reset  InitialOutput=0
  "tau_fl_agree " : Outport  Port=2  OutputWhenDisabled=reset  InitialOutput=0
  tau_ar_agree : Outport  Port=3  OutputWhenDisabled=reset  InitialOutput=0
  tau_al_agree : Outport  Port=4  OutputWhenDisabled=reset  InitialOutput=0
  wires:
  AND3/1 -> tau_al_agree/1
  Data Store Read3/1 -> Plus7/1, Plus6/1
  Constant6/1 -> Gain6/1
  Gain6/1 -> Plus6/2
  Plus6/1 -> GreaterThan7/2
  Data Store Read7/1 -> GreaterThan6/1, GreaterThan7/1
  Constant7/1 -> Gain7/1
  Gain7/1 -> Plus7/2
  Plus7/1 -> GreaterThan6/2
  GreaterThan7/1 -> AND3/1
  GreaterThan6/1 -> AND3/2
  AND2/1 -> tau_ar_agree/1
  GreaterThan4/1 -> AND2/2
  GreaterThan5/1 -> AND2/1
  Plus5/1 -> GreaterThan4/2
  Gain5/1 -> Plus5/2
  Constant5/1 -> Gain5/1
  Data Store Read6/1 -> GreaterThan5/1, GreaterThan4/1
  Plus4/1 -> GreaterThan5/2
  Gain4/1 -> Plus4/2
  Constant4/1 -> Gain4/1
  Data Store Read2/1 -> Plus4/1, Plus5/1
  AND1/1 -> "tau_fl_agree "/1
  Data Store Read1/1 -> Plus3/1, Plus2/1
  Constant2/1 -> Gain2/1
  Gain2/1 -> Plus2/2
  Plus2/1 -> GreaterThan3/2
  Data Store Read5/1 -> GreaterThan2/1, GreaterThan3/1
  Constant3/1 -> Gain3/1
  Gain3/1 -> Plus3/2
  Plus3/1 -> GreaterThan2/2
  GreaterThan3/1 -> AND1/1
  GreaterThan2/1 -> AND1/2
  AND/1 -> tau_fr_agree/1
  GreaterThan/1 -> AND/2
  GreaterThan1/1 -> AND/1
  Plus1/1 -> GreaterThan/2
  Gain1/1 -> Plus1/2
  Constant1/1 -> Gain1/1
  Data Store Read4/1 -> GreaterThan1/1, GreaterThan/1
  Plus/1 -> GreaterThan1/2
  Gain/1 -> Plus/2
  Constant/1 -> Gain/1
  Data Store Read/1 -> Plus/1, Plus1/1

== system HANcoder_E407_TTA_Controller_v4_5/HANcoder STM32 Target - E407-STM32 algorithm/TTA CAN System/TTA System/Matrix Cycle Manager/Backup Board Matrix Cycle/Backup board basic cycle 1/COMP Task - MF/MF_main/Agreement between Out2 and out3 ==
  Enable : EnablePort
  AND{,1..3} (4 alike) : Logic  IconShape=distinctive  AllPortsSameDT=off  OutDataTypeStr=boolean
  Constant{,1..7} (8 alike) : Constant  Value=tau_range
  Data Store Read : DataStoreRead  DataStoreName=tau_fr_out2
  Data Store Read1 : DataStoreRead  DataStoreName=tau_fl_out2
  Data Store Read2 : DataStoreRead  DataStoreName=tau_ar_out2
  Data Store Read3 : DataStoreRead  DataStoreName=tau_al_out2
  Data Store Read4 : DataStoreRead  DataStoreName=tau_fr_out3
  Data Store Read5 : DataStoreRead  DataStoreName=tau_fl_out3
  Data Store Read6 : DataStoreRead  DataStoreName=tau_ar_out3
  Data Store Read7 : DataStoreRead  DataStoreName=tau_al_out3
  Gain{,1..7} (8 alike) : Gain  Gain=e_width
  GreaterThan{,2,4,6} (4 alike) : RelationalOperator  OutDataTypeStr=boolean  RndMeth=Simplest
  GreaterThan{1,3,5,7} (4 alike) : RelationalOperator  Operator=<=  OutDataTypeStr=boolean  RndMeth=Simplest
  Plus{,2,4,6} (4 alike) : Sum
  Plus{1,3,5,7} (4 alike) : Sum  Inputs=+-
  tau_fr_agree : Outport  OutputWhenDisabled=reset  InitialOutput=0
  "tau_fl_agree " : Outport  Port=2  OutputWhenDisabled=reset  InitialOutput=0
  tau_ar_agree : Outport  Port=3  OutputWhenDisabled=reset  InitialOutput=0
  tau_al_agree : Outport  Port=4  OutputWhenDisabled=reset  InitialOutput=0
  wires:
  Data Store Read/1 -> Plus1/1, Plus/1
  Constant/1 -> Gain/1
  Gain/1 -> Plus/2
  Plus/1 -> GreaterThan1/2
  Data Store Read4/1 -> GreaterThan/1, GreaterThan1/1
  Constant1/1 -> Gain1/1
  Gain1/1 -> Plus1/2
  Plus1/1 -> GreaterThan/2
  GreaterThan1/1 -> AND/1
  GreaterThan/1 -> AND/2
  AND/1 -> tau_fr_agree/1
  GreaterThan2/1 -> AND1/2
  GreaterThan3/1 -> AND1/1
  Plus3/1 -> GreaterThan2/2
  Gain3/1 -> Plus3/2
  Constant3/1 -> Gain3/1
  Data Store Read5/1 -> GreaterThan3/1, GreaterThan2/1
  Plus2/1 -> GreaterThan3/2
  Gain2/1 -> Plus2/2
  Constant2/1 -> Gain2/1
  Data Store Read1/1 -> Plus2/1, Plus3/1
  AND1/1 -> "tau_fl_agree "/1
  Data Store Read2/1 -> Plus5/1, Plus4/1
  Constant4/1 -> Gain4/1
  Gain4/1 -> Plus4/2
  Plus4/1 -> GreaterThan5/2
  Data Store Read6/1 -> GreaterThan4/1, GreaterThan5/1
  Constant5/1 -> Gain5/1
  Gain5/1 -> Plus5/2
  Plus5/1 -> GreaterThan4/2
  GreaterThan5/1 -> AND2/1
  GreaterThan4/1 -> AND2/2
  AND2/1 -> tau_ar_agree/1
  GreaterThan6/1 -> AND3/2
  GreaterThan7/1 -> AND3/1
  Plus7/1 -> GreaterThan6/2
  Gain7/1 -> Plus7/2
  Constant7/1 -> Gain7/1
  Data Store Read7/1 -> GreaterThan7/1, GreaterThan6/1
  Plus6/1 -> GreaterThan7/2
  Gain6/1 -> Plus6/2
  Constant6/1 -> Gain6/1
  Data Store Read3/1 -> Plus6/1, Plus7/1
  AND3/1 -> tau_al_agree/1

== system HANcoder_E407_TTA_Controller_v4_5/HANcoder STM32 Target - E407-STM32 algorithm/TTA CAN System/TTA System/Matrix Cycle Manager/Backup Board Matrix Cycle/Backup board basic cycle 1/COMP Task - MF/MF_main/Agreement between out1 and out2 ==
  Enable : EnablePort
  AND{,1..3} (4 alike) : Logic  IconShape=distinctive  AllPortsSameDT=off  OutDataTypeStr=boolean
  Constant{,1..7} (8 alike) : Constant  Value=tau_range
  Data Store Read : DataStoreRead  DataStoreName=tau_fr_out1
  Data Store Read1 : DataStoreRead  DataStoreName=tau_fl_out1
  Data Store Read2 : DataStoreRead  DataStoreName=tau_ar_out1
  Data Store Read3 : DataStoreRead  DataStoreName=tau_al_out1
  Data Store Read4 : DataStoreRead  DataStoreName=tau_fr_out2
  Data Store Read5 : DataStoreRead  DataStoreName=tau_fl_out2
  Data Store Read6 : DataStoreRead  DataStoreName=tau_ar_out2
  Data Store Read7 : DataStoreRead  DataStoreName=tau_al_out2
  Gain{,1..7} (8 alike) : Gain  Gain=e_width
  GreaterThan{,2,4,6} (4 alike) : RelationalOperator  OutDataTypeStr=boolean  RndMeth=Simplest
  GreaterThan{1,3,5,7} (4 alike) : RelationalOperator  Operator=<=  OutDataTypeStr=boolean  RndMeth=Simplest
  Plus{,2,4,6} (4 alike) : Sum
  Plus{1,3,5,7} (4 alike) : Sum  Inputs=+-
  tau_fr_agree : Outport  OutputWhenDisabled=reset  InitialOutput=0
  "tau_fl_agree " : Outport  Port=2  OutputWhenDisabled=reset  InitialOutput=0
  tau_ar_agree : Outport  Port=3  OutputWhenDisabled=reset  InitialOutput=0
  tau_al_agree : Outport  Port=4  OutputWhenDisabled=reset  InitialOutput=0
  wires:
  AND3/1 -> tau_al_agree/1
  Data Store Read3/1 -> Plus7/1, Plus6/1
  Constant6/1 -> Gain6/1
  Gain6/1 -> Plus6/2
  Plus6/1 -> GreaterThan7/2
  Data Store Read7/1 -> GreaterThan6/1, GreaterThan7/1
  Constant7/1 -> Gain7/1
  Gain7/1 -> Plus7/2
  Plus7/1 -> GreaterThan6/2
  GreaterThan7/1 -> AND3/1
  GreaterThan6/1 -> AND3/2
  AND2/1 -> tau_ar_agree/1
  GreaterThan4/1 -> AND2/2
  GreaterThan5/1 -> AND2/1
  Plus5/1 -> GreaterThan4/2
  Gain5/1 -> Plus5/2
  Constant5/1 -> Gain5/1
  Data Store Read6/1 -> GreaterThan5/1, GreaterThan4/1
  Plus4/1 -> GreaterThan5/2
  Gain4/1 -> Plus4/2
  Constant4/1 -> Gain4/1
  Data Store Read2/1 -> Plus4/1, Plus5/1
  AND1/1 -> "tau_fl_agree "/1
  Data Store Read1/1 -> Plus3/1, Plus2/1
  Constant2/1 -> Gain2/1
  Gain2/1 -> Plus2/2
  Plus2/1 -> GreaterThan3/2
  Data Store Read5/1 -> GreaterThan2/1, GreaterThan3/1
  Constant3/1 -> Gain3/1
  Gain3/1 -> Plus3/2
  Plus3/1 -> GreaterThan2/2
  GreaterThan3/1 -> AND1/1
  GreaterThan2/1 -> AND1/2
  AND/1 -> tau_fr_agree/1
  GreaterThan/1 -> AND/2
  GreaterThan1/1 -> AND/1
  Plus1/1 -> GreaterThan/2
  Gain1/1 -> Plus1/2
  Constant1/1 -> Gain1/1
  Data Store Read4/1 -> GreaterThan1/1, GreaterThan/1
  Plus/1 -> GreaterThan1/2
  Gain/1 -> Plus/2
  Constant/1 -> Gain/1
  Data Store Read/1 -> Plus/1, Plus1/1

== system HANcoder_E407_TTA_Controller_v4_5/HANcoder STM32 Target - E407-STM32 algorithm/TTA CAN System/TTA System/Matrix Cycle Manager/Backup Board Matrix Cycle/Backup board basic cycle 1/COMP Task - MF/MF_main/Subsystem ==
  Action Port : Inport
  Action Port1 : Inport  Port=2
  Action Port2 : Inport  Port=3
  If Action Subsystem : Subsystem  TreatAsAtomicUnit=on
  If Action Subsystem1 : Subsystem  TreatAsAtomicUnit=on
  If Action Subsystem2 : Subsystem  TreatAsAtomicUnit=on
  wires:
  Action Port2/1 -> If Action Subsystem2/Action
  Action Port/1 -> If Action Subsystem/Action
  Action Port1/1 -> If Action Subsystem1/Action

== system HANcoder_E407_TTA_Controller_v4_5/HANcoder STM32 Target - E407-STM32 algorithm/TTA CAN System/TTA System/Matrix Cycle Manager/Backup Board Matrix Cycle/Backup board basic cycle 1/COMP Task - Rx_Output_Control1_Check/Process_Messages/Demux message CAN1 and check coherence ==
  CAN1_Rx_msg : Inport  OutDataTypeStr=Bus: msg_buffer_type
  expected_board_id : Inport  Port=2
  Enable : EnablePort
  Bus Creator : BusCreator  Inputs=8  OutDataTypeStr=Bus: msg_buffer_type
  Bus Selector : BusSelector  OutputSignals=Buffer_1,Buffer_2,Buffer_3,Buffer_4,Buffer_5,Buffer_6,Buffer_7,Buffer_8
  Constant : Constant  Value=0  OutDataTypeStr=uint8
  Equal : RelationalOperator  Operator===  OutDataTypeStr=boolean  RndMeth=Simplest
  Subsystem : Subsystem
  Terminator : Terminator
  msg_count>2_DEBUG : Subsystem
  CAN1_msg : Outport  OutDataTypeStr=Bus: msg_buffer_type
  Msg_Count_CAN1 : Outport  Port=2
  CAN1_msg_coherent : Outport  Port=3  OutputWhenDisabled=reset  InitialOutput=0
  wires:
  Subsystem/1(basic_cycle) -> Terminator/1
  Constant/1 -> Bus Creator/1
  Bus Creator/1 -> CAN1_msg/1
  Subsystem/2(msg_count) -> Msg_Count_CAN1/1, msg_count>2_DEBUG/1(msg_c)
  Bus Selector/1 -> Subsystem/1(Msg_Temporal_Data)  "<Buffer_1>"
  Subsystem/3(board_id) -> Equal/1
  Bus Selector/4 -> Bus Creator/4  "<Buffer_4>"
  Bus Selector/8 -> Bus Creator/8  "<Buffer_8>"
  Bus Selector/7 -> Bus Creator/7  "<Buffer_7>"
  Bus Selector/5 -> Bus Creator/5  "<Buffer_5>"
  Bus Selector/6 -> Bus Creator/6  "<Buffer_6>"
  expected_board_id/1 -> Equal/2
  Equal/1 -> CAN1_msg_coherent/1
  CAN1_Rx_msg/1 -> Bus Selector/1
  Bus Selector/3 -> Bus Creator/3  "<Buffer_3>"
  Bus Selector/2 -> Bus Creator/2  "<Buffer_2>"

== system HANcoder_E407_TTA_Controller_v4_5/HANcoder STM32 Target - E407-STM32 algorithm/TTA CAN System/TTA System/Matrix Cycle Manager/Backup Board Matrix Cycle/Backup board basic cycle 1/COMP Task - Rx_Output_Control1_Check/Process_Messages/Demux message CAN1 and check coherence1 ==
  CAN2_Rx_msg : Inport  OutDataTypeStr=Bus: msg_buffer_type
  expected_board_id : Inport  Port=2
  Enable : EnablePort
  Bus Creator : BusCreator  Inputs=8  OutDataTypeStr=Bus: msg_buffer_type
  Bus Selector : BusSelector  OutputSignals=Buffer_1,Buffer_2,Buffer_3,Buffer_4,Buffer_5,Buffer_6,Buffer_7,Buffer_8
  Constant : Constant  Value=0  OutDataTypeStr=uint8
  Equal : RelationalOperator  Operator===  OutDataTypeStr=boolean  RndMeth=Simplest
  Subsystem : Subsystem
  Terminator : Terminator
  msg_count>2_DEBUG : Subsystem
  CAN2_msg_coherent : Outport  OutputWhenDisabled=reset  InitialOutput=0
  Msg_Count_CAN2 : Outport  Port=2
  CAN2_msg : Outport  Port=3  OutDataTypeStr=Bus: msg_buffer_type
  wires:
  Subsystem/1(basic_cycle) -> Terminator/1
  Constant/1 -> Bus Creator/1
  Bus Creator/1 -> CAN2_msg/1
  Subsystem/2(msg_count) -> Msg_Count_CAN2/1, msg_count>2_DEBUG/1(msg_c)
  Bus Selector/1 -> Subsystem/1(Msg_Temporal_Data)  "<Buffer_1>"
  Subsystem/3(board_id) -> Equal/1
  Bus Selector/4 -> Bus Creator/4  "<Buffer_4>"
  Bus Selector/8 -> Bus Creator/8  "<Buffer_8>"
  Bus Selector/7 -> Bus Creator/7  "<Buffer_7>"
  Bus Selector/5 -> Bus Creator/5  "<Buffer_5>"
  Bus Selector/6 -> Bus Creator/6  "<Buffer_6>"
  expected_board_id/1 -> Equal/2
  Equal/1 -> CAN2_msg_coherent/1
  CAN2_Rx_msg/1 -> Bus Selector/1
  Bus Selector/3 -> Bus Creator/3  "<Buffer_3>"
  Bus Selector/2 -> Bus Creator/2  "<Buffer_2>"

== system HANcoder_E407_TTA_Controller_v4_5/HANcoder STM32 Target - E407-STM32 algorithm/TTA CAN System/TTA System/Matrix Cycle Manager/Backup Board Matrix Cycle/Backup board basic cycle 1/COMP Task - Rx_Output_Control2_Check/Process_Messages/Demux message CAN1 and check coherence ==
  CAN1_Rx_msg : Inport  OutDataTypeStr=Bus: msg_buffer_type
  expected_board_id : Inport  Port=2
  Enable : EnablePort
  Bus Creator : BusCreator  Inputs=8  OutDataTypeStr=Bus: msg_buffer_type
  Bus Selector : BusSelector  OutputSignals=Buffer_1,Buffer_2,Buffer_3,Buffer_4,Buffer_5,Buffer_6,Buffer_7,Buffer_8
  Constant : Constant  Value=0  OutDataTypeStr=uint8
  Equal : RelationalOperator  Operator===  OutDataTypeStr=boolean  RndMeth=Simplest
  Subsystem : Subsystem
  Terminator : Terminator
  msg_count>2_DEBUG : Subsystem
  CAN1_msg : Outport  OutDataTypeStr=Bus: msg_buffer_type
  Msg_Count_CAN1 : Outport  Port=2
  CAN1_msg_coherent : Outport  Port=3  OutputWhenDisabled=reset  InitialOutput=0
  wires:
  Bus Selector/2 -> Bus Creator/2  "<Buffer_2>"
  Bus Selector/3 -> Bus Creator/3  "<Buffer_3>"
  CAN1_Rx_msg/1 -> Bus Selector/1
  Equal/1 -> CAN1_msg_coherent/1
  expected_board_id/1 -> Equal/2
  Bus Selector/6 -> Bus Creator/6  "<Buffer_6>"
  Bus Selector/5 -> Bus Creator/5  "<Buffer_5>"
  Bus Selector/7 -> Bus Creator/7  "<Buffer_7>"
  Bus Selector/8 -> Bus Creator/8  "<Buffer_8>"
  Bus Selector/4 -> Bus Creator/4  "<Buffer_4>"
  Subsystem/3(board_id) -> Equal/1
  Bus Selector/1 -> Subsystem/1(Msg_Temporal_Data)  "<Buffer_1>"
  Subsystem/2(msg_count) -> msg_count>2_DEBUG/1(msg_c), Msg_Count_CAN1/1
  Bus Creator/1 -> CAN1_msg/1
  Constant/1 -> Bus Creator/1
  Subsystem/1(basic_cycle) -> Terminator/1

== system HANcoder_E407_TTA_Controller_v4_5/HANcoder STM32 Target - E407-STM32 algorithm/TTA CAN System/TTA System/Matrix Cycle Manager/Backup Board Matrix Cycle/Backup board basic cycle 1/COMP Task - Rx_Output_Control2_Check/Process_Messages/Demux message CAN1 and check coherence1 ==
  CAN2_Rx_msg : Inport  OutDataTypeStr=Bus: msg_buffer_type
  expected_board_id : Inport  Port=2
  Enable : EnablePort
  Bus Creator : BusCreator  Inputs=8  OutDataTypeStr=Bus: msg_buffer_type
  Bus Selector : BusSelector  OutputSignals=Buffer_1,Buffer_2,Buffer_3,Buffer_4,Buffer_5,Buffer_6,Buffer_7,Buffer_8
  Constant : Constant  Value=0  OutDataTypeStr=uint8
  Equal : RelationalOperator  Operator===  OutDataTypeStr=boolean  RndMeth=Simplest
  Subsystem : Subsystem
  Terminator : Terminator
  msg_count>2_DEBUG : Subsystem
  CAN2_msg_coherent : Outport  OutputWhenDisabled=reset  InitialOutput=0
  Msg_Count_CAN2 : Outport  Port=2
  CAN2_msg : Outport  Port=3  OutDataTypeStr=Bus: msg_buffer_type
  wires:
  Bus Selector/2 -> Bus Creator/2  "<Buffer_2>"
  Bus Selector/3 -> Bus Creator/3  "<Buffer_3>"
  CAN2_Rx_msg/1 -> Bus Selector/1
  Equal/1 -> CAN2_msg_coherent/1
  expected_board_id/1 -> Equal/2
  Bus Selector/6 -> Bus Creator/6  "<Buffer_6>"
  Bus Selector/5 -> Bus Creator/5  "<Buffer_5>"
  Bus Selector/7 -> Bus Creator/7  "<Buffer_7>"
  Bus Selector/8 -> Bus Creator/8  "<Buffer_8>"
  Bus Selector/4 -> Bus Creator/4  "<Buffer_4>"
  Subsystem/3(board_id) -> Equal/1
  Bus Selector/1 -> Subsystem/1(Msg_Temporal_Data)  "<Buffer_1>"
  Subsystem/2(msg_count) -> msg_count>2_DEBUG/1(msg_c), Msg_Count_CAN2/1
  Bus Creator/1 -> CAN2_msg/1
  Constant/1 -> Bus Creator/1
  Subsystem/1(basic_cycle) -> Terminator/1

== system HANcoder_E407_TTA_Controller_v4_5/HANcoder STM32 Target - E407-STM32 algorithm/TTA CAN System/TTA System/Matrix Cycle Manager/Backup Board Matrix Cycle/Backup board basic cycle 1/COMP Task - Rx_Output_Master_Check/OutputControl1 Tx condition2/Switch Case Action Subsystem ==
  In1 : Inport
  Action Port : ActionPort  ActionType=then
  Out1 : Outport
  wires:
  In1/1 -> Out1/1
